simulink model "Hinf"  (R2022a)
settings: Solver=VariableStepAuto  StartTime=0.0  StopTime=0.2  RelTol=1e-3
values from neighbouring files (symbols this model uses):
  d0 = 1e-09    [system_parameters.mat]    (also in system_parameters_3d.mat)
  fs = 30000    [system_parameters.mat]    (also in system_parameters_3d.mat = 20000)
  g = 0.0011    [system_parameters.mat]    (also in system_parameters_3d.mat)
  Ga = 1.2e-09    [system_parameters.mat]
  Gc = 1000000000    [system_parameters.mat]    (also in system_parameters_3d.mat)
  Gv = 15    [system_parameters.mat]    (also in system_parameters_3d.mat)
  k = 2.29    [hinf_design.m]    (also in system_parameters.mat = 16500000000; system_parameters_3d.mat = 16500000000)
  vb = 1.025    [system_parameters.mat]    (also in system_parameters_3d.mat)
  wa = 120000    [hinf_design.m]    (also in system_parameters.mat)
  wc = 13000    [system_parameters.mat]    (also in system_parameters_3d.mat)
  wv = 4000    [hinf_design.m]    (also in system_parameters.mat; system_parameters_3d.mat)
  zeta = 0.9    [system_parameters.mat]
libraries: simulink x1
settings Model: Creator=doamarar  LastModifiedBy=doamarar

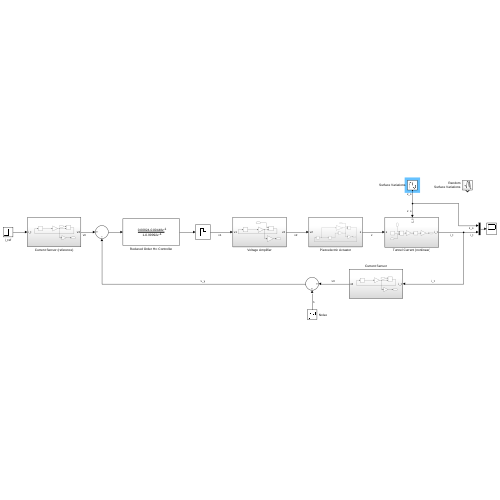
[thumbnail: Simulink's stored preview of the top-level diagram]
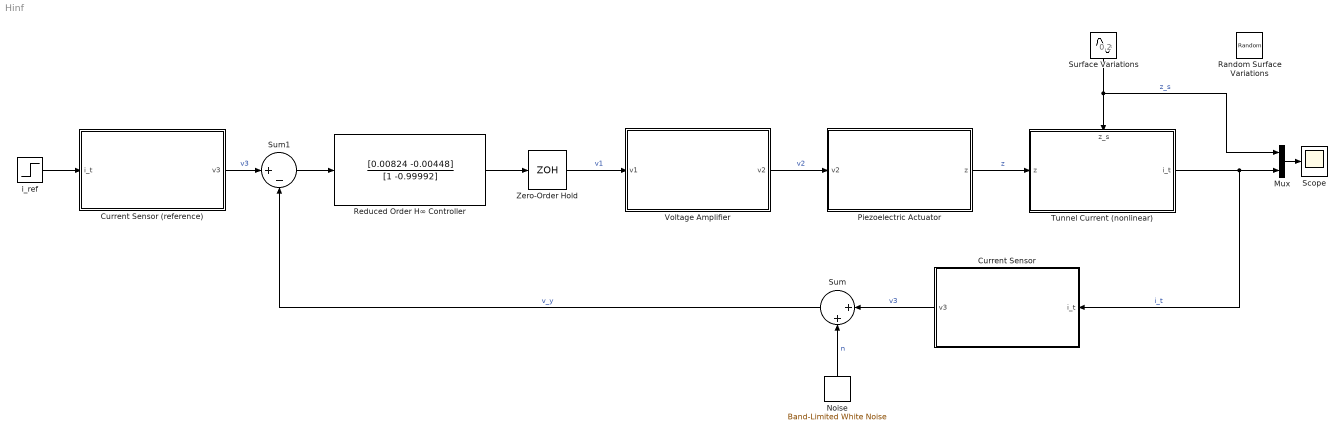
== system Hinf ==
  note: 0.2
  Current Sensor : Subsystem
  Current Sensor (reference) : Subsystem
  Mux : Mux  Inputs=2
  Noise : simulink/Sources/Band-Limited White Noise  Cov=[0.000000001]  Ts=1/fs  seed=[23341]
  Piezoelectric Actuator : Subsystem
  Random Surface Variations : RandomNumber  Variance=2*10^-25  SampleTime=0.0000333333
  Reduced Order H∞ Controller : DiscreteFilter  Numerator=[0.00824 -0.00448]  Denominator=[1 -0.99992]  SampleTime=1/fs
  Scope : Scope
  Sum : Sum  Inputs=|++
  Sum1 : Sum  Inputs=|+-
  Surface Variations : Sin  Amplitude=5*10^-11  Frequency=600  SampleTime=1/fs
  Tunnel Current (nonlinear) : Subsystem
      settings: PortSchema="{\"entries\":[{\"content\":{\"sides\":[{\"content\":{\"connectorIds\":[\"In1\"]},\"type\":\"ConnectorPlacement.EquallySpacedRectSide\",\"uuid\":\"147d123d-45a5-4220-b41f-835da98fb0cd\"},{\"content\":{\"connectorIds\":[\"Out1\"],\"side\":\"RIGHT\"},\"type\":\"ConnectorPlacement.EquallySpacedRectSide\",\"uuid\":\"1a05abba-b8fc-4d61-92c8-15761dd3dd6b\"},{\"content\":{\"connectorIds\":[\"In2\"],\"side\":\"TOP\"},\"type\":\"ConnectorPlacement.EquallySpacedRectSide\",\"uuid\":\"bc9d4ee1-4dd7-4150-9ece-b291902d4347\"}]},\"type\":\"ConnectorPlacement.EquallySpacedConnector\",\"uuid\":\"916abd9f-079e-4be3-a864-fdb35439c6f4\"}],\"packageUris\":[\"http://schema.mathworks.com/mf0/Connector/R2020b\"],\"version\":\"1.0\"}"
  Voltage Amplifier : Subsystem
  Zero-Order Hold : ZeroOrderHold  SampleTime=1/fs
  i_ref : Step  Time=0  After=0.5*10^-9  SampleTime=1/fs
  wires:
  Tunnel Current (nonlinear)/1(i_t) -> Mux/2, Current Sensor/1(i_t)  "i_t"
  i_ref/1 -> Current Sensor (reference)/1(i_t)
  Sum1/1 -> Reduced Order H∞ Controller/1
  Voltage Amplifier/1(v2) -> Piezoelectric Actuator/1(v2)  "v2"
  Piezoelectric Actuator/1(z) -> Tunnel Current (nonlinear)/1(z)  "z"
  Reduced Order H∞ Controller/1 -> Zero-Order Hold/1
  Surface Variations/1 -> Mux/1, Tunnel Current (nonlinear)/2(z_s)  "z_s"
  Current Sensor/1(v3) -> Sum/1  "v3"
  Noise/1 -> Sum/2  "n"
  Sum/1 -> Sum1/2  "v_y"
  Zero-Order Hold/1 -> Voltage Amplifier/1(v1)  "v1"
  Current Sensor (reference)/1(v3) -> Sum1/1  "v3"
  Mux/1 -> Scope/1

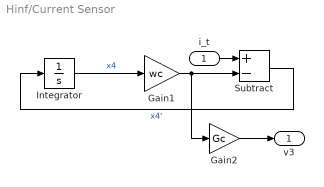
== system Hinf/Current Sensor ==
  i_t : Inport
  Gain1 : Gain  Gain=wc
  Gain2 : Gain  Gain=Gc
  Integrator : Integrator
  Subtract : Sum  Inputs=+-
  v3 : Outport
  wires:
  Gain2/1 -> v3/1
  Integrator/1 -> Gain1/1  "x4"
  Gain1/1 -> Gain2/1, Subtract/2
  i_t/1 -> Subtract/1
  Subtract/1 -> Integrator/1  "x4'"

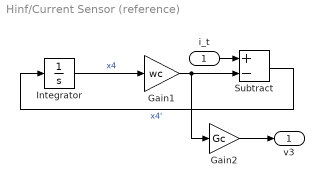
== system Hinf/Current Sensor (reference) ==
  i_t : Inport
  Gain1 : Gain  Gain=wc
  Gain2 : Gain  Gain=Gc
  Integrator : Integrator
  Subtract : Sum  Inputs=+-
  v3 : Outport
  wires:
  Gain2/1 -> v3/1
  Integrator/1 -> Gain1/1  "x4"
  Gain1/1 -> Gain2/1, Subtract/2
  i_t/1 -> Subtract/1
  Subtract/1 -> Integrator/1  "x4'"

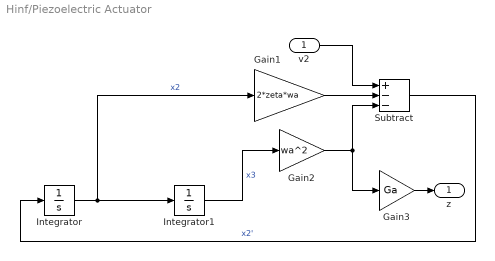
== system Hinf/Piezoelectric Actuator ==
  v2 : Inport
  Gain1 : Gain  Gain=2*zeta*wa
  Gain2 : Gain  Gain=wa^2
  Gain3 : Gain  Gain=Ga
  Integrator : Integrator
  Integrator1 : Integrator
  Subtract : Sum  Inputs=+--
  z : Outport
  wires:
  Subtract/1 -> Integrator/1  "x2'"
  Gain1/1 -> Subtract/2
  v2/1 -> Subtract/1
  Gain2/1 -> Gain3/1, Subtract/3
  Integrator/1 -> Gain1/1, Integrator1/1  "x2"
  Gain3/1 -> z/1
  Integrator1/1 -> Gain2/1  "x3"

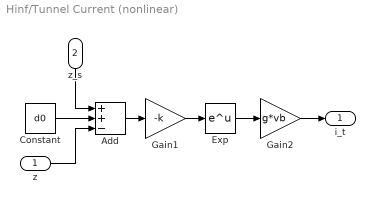
== system Hinf/Tunnel Current (nonlinear) ==
  z : Inport
  z_s : Inport  Port=2
  Add : Sum  Inputs=++-
  Constant : Constant  Value=d0
  Exp : Math
  Gain1 : Gain  Gain=-k
  Gain2 : Gain  Gain=g*vb
  i_t : Outport
  wires:
  Add/1 -> Gain1/1
  z_s/1 -> Add/1
  z/1 -> Add/3
  Gain1/1 -> Exp/1
  Exp/1 -> Gain2/1
  Gain2/1 -> i_t/1
  Constant/1 -> Add/2

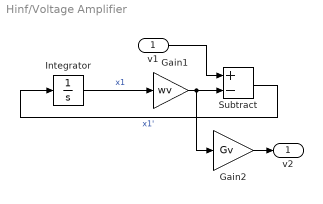
== system Hinf/Voltage Amplifier ==
  v1 : Inport
  Gain1 : Gain  Gain=wv
  Gain2 : Gain  Gain=Gv
  Integrator : Integrator
  Subtract : Sum  Inputs=+-
  v2 : Outport
  wires:
  Integrator/1 -> Gain1/1  "x1"
  Subtract/1 -> Integrator/1  "x1'"
  Gain1/1 -> Gain2/1, Subtract/2
  Gain2/1 -> v2/1
  v1/1 -> Subtract/1
